simulink model "simulink_group8_2_serial_"  (R2020a)
settings: Solver=FixedStepAuto  StartTime=0.0  StopTime=40  FixedStep=1e-3  RelTol=1e-3  EnableMultiTasking=on
undefined symbols (not defined in the file): A0, A1, D0, D1, D10, D11, D12, D13, D2, D3, D4, D5, D6, D7, D8, D9, magnitude, PTA0, PTA1, PTA2, PTB2, PTB23, PTB3, PTB9, PTC16, PTC17, PTC2, PTC3, PTC4, PTD0, PTD1, PTD2, PTD3
libraries: frdmk64flib x20, etargetslib x10, simulink x4
settings Model: ExtModeTrigDuration=5  Creator=namby  LastModifiedBy=bacTh
settings SolverCC: AutoInsertRateTranBlk=on
settings OptimizationCC: EnhancedBackFolding=on  PassReuseOutputArgsAs=Individual arguments  ZeroExternalMemoryAtStartup=off  ZeroInternalMemoryAtStartup=off  MaxStackSize=64  OptimizeBlockOrder=speed  DifferentSizesBufferReuse=on  OptimizationCustomize=off  EfficientTunableParamExpr=on
settings DebuggingCC: ParameterTunabilityLossMsg=error
settings HardwareCC: ProdBitPerPointer=32  ProdBitPerSizeT=32  ProdBitPerPtrDiffT=32  ProdLargestAtomicInteger=Long  ProdLargestAtomicFloat=Double  ProdWordSize=32  ProdHWDeviceType=ARM Compatible->ARM Cortex
settings SFSimCC: MATLABDynamicMemAlloc=off
settings RTWCC: SystemTargetFile=ert.tlc  HardwareBoard=NXP FRDM-K64F  TemplateMakefile=ert_default_tmf  Toolchain=GNU Tools for ARM Embedded Processors
settings CodeAppCC: ForceParamTrailComments=on  IgnoreCustomStorageClasses=off  OperatorAnnotations=on  SimulinkDataObjDesc=on  SFDataObjDesc=on  InsertBlockDesc=on
settings ConfigComp: CovBoundaryAbsTol=1.0e-5
settings SettingsController: UseSoCProfilerForTargets=0

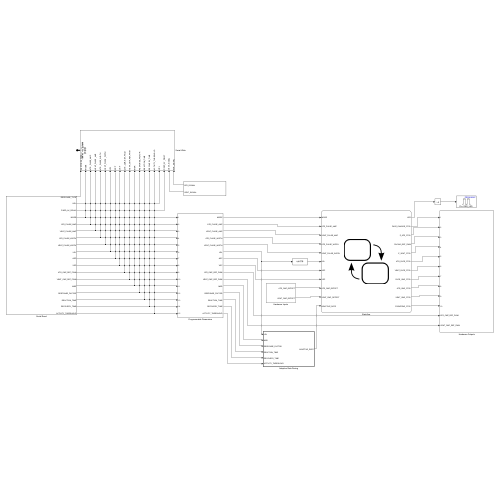
[thumbnail: Simulink's stored preview of the top-level diagram]
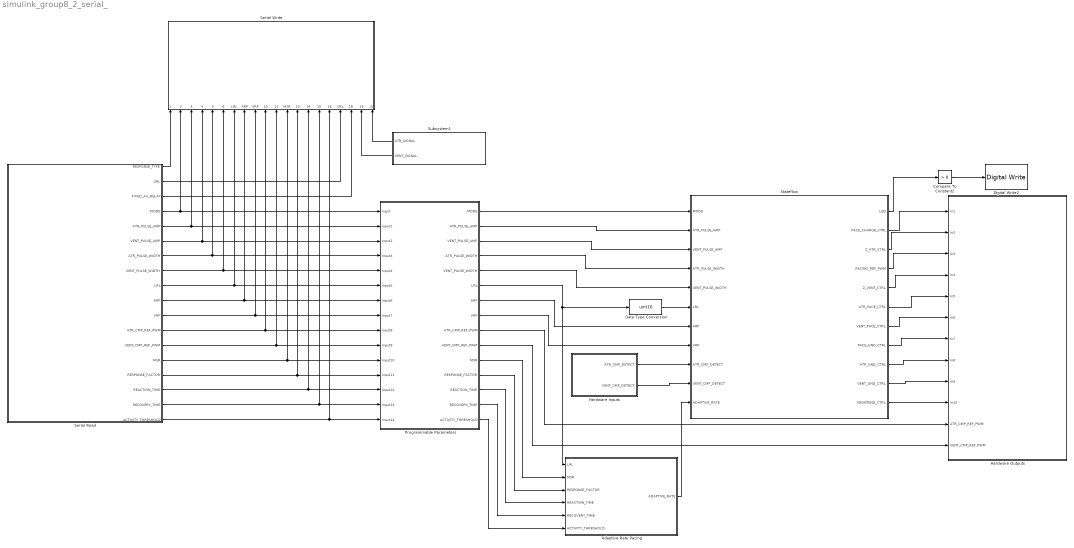
== system simulink_group8_2_serial_ ==
  Adaptive Rate Pacing : Subsystem  TreatAsAtomicUnit=on
  Compare To Constant2 : simulink/Logic and Bit Operations/Compare To Constant  relop=>  const=0  OutDataTypeStr=boolean
  Data Type Conversion : DataTypeConversion  OutDataTypeStr=uint16
  Digital Write2 : frdmk64flib/Digital Write  Whichpin=RED_LED
  Hardware Inputs : Subsystem
  Hardware Outputs : Subsystem
  Programmable Parameters : Subsystem
  Serial Read : Subsystem
  Serial Write : Subsystem
  Stateflow : Stateflow chart  TreatAsAtomicUnit=on
      settings: PortSchema="{\"entries\":[{\"content\":{\"sides\":[{\"content\":{\"connectorIds\":[\"In1\",\"In2\",\"In3\",\"In4\",\"In5\",\"In6\",\"In7\",\"In8\",\"In9\",\"In10\",\"In11\"]},\"type\":\"ConnectorPlacement.EquallySpacedRectSide\",\"uuid\":\"4861ea68-cca1-4690-bebf-db066e06f2bf\"},{\"content\":{\"connectorIds\":[\"Out11\",\"Out1\",\"Out2\",\"Out3\",\"Out4\",\"Out5\",\"Out6\",\"Out7\",\"Out8\",\"Out9\",\"Out10\"],\"side\":\"RIGHT\"},\"type\":\"ConnectorPlacement.EquallySpacedRectSide\",\"uuid\":\"4fa1417b-a578-4dd5-8ec9-8fcbce219e5e\"},{\"content\":{\"side\":\"TOP\"},\"type\":\"ConnectorPlacement.EquallySpacedRectSide\",\"uuid\":\"410f88ae-5c1c-4ed5-8b61-d3fe3ab7a61c\"}]},\"type\":\"ConnectorPlacement.EquallySpacedConnector\",\"uuid\":\"8afcebbc-da82-4773-8c00-253856c85373\"}],\"packageUris\":[\"http://schema.mathworks.com/mf0/Connector/R2020b\"],\"version\":\"1.0\"}"
  Subsystem1 : Subsystem
  wires:
  Programmable Parameters/1(MODE) -> Stateflow/1(MODE)
  Programmable Parameters/2(ATR_PULSE_AMP) -> Stateflow/2(ATR_PULSE_AMP)
  Programmable Parameters/3(VENT_PULSE_AMP) -> Stateflow/3(VENT_PULSE_AMP)
  Programmable Parameters/4(ATR_PULSE_WIDTH) -> Stateflow/4(ATR_PULSE_WIDTH)
  Programmable Parameters/5(VENT_PULSE_WIDTH) -> Stateflow/5(VENT_PULSE_WIDTH)
  Programmable Parameters/6(LRL) -> Adaptive Rate Pacing/1(LRL), Data Type Conversion/1
  Programmable Parameters/7(ARP) -> Stateflow/7(ARP)
  Programmable Parameters/8(VRP) -> Stateflow/8(VRP)
  Hardware Inputs/1(ATR_CMP_DETECT) -> Stateflow/9(ATR_CMP_DETECT)
  Hardware Inputs/2(VENT_CMP_DETECT) -> Stateflow/10(VENT_CMP_DETECT)
  Stateflow/1(PACE_CHARGE_CTRL) -> Hardware Outputs/1(In1)
  Stateflow/2(Z_ATR_CTRL) -> Hardware Outputs/2(In2)
  Stateflow/3(PACING_REF_PWM) -> Hardware Outputs/3(In3)
  Stateflow/4(Z_VENT_CTRL) -> Hardware Outputs/4(In4)
  Stateflow/5(ATR_PACE_CTRL) -> Hardware Outputs/5(In5)
  Stateflow/6(VENT_PACE_CTRL) -> Hardware Outputs/6(In6)
  Stateflow/7(PACE_GND_CTRL) -> Hardware Outputs/7(In7)
  Stateflow/8(ATR_GND_CTRL) -> Hardware Outputs/8(In8)
  Stateflow/9(VENT_GND_CTRL) -> Hardware Outputs/9(In9)
  Stateflow/10(FRONTEND_CTRL) -> Hardware Outputs/10(In10)
  Programmable Parameters/9(ATR_CMP_REF_PWM) -> Hardware Outputs/11(ATR_CMP_REF_PWM)
  Programmable Parameters/10(VENT_CMP_REF_PWM) -> Hardware Outputs/12(VENT_CMP_REF_PWM)
  Adaptive Rate Pacing/1(ADAPTIVE_RATE) -> Stateflow/11(ADAPTIVE_RATE)
  Programmable Parameters/15(ACTIVITY_THRESHOLD) -> Adaptive Rate Pacing/6(ACTIVITY_THRESHOLD)
  Programmable Parameters/13(REACTION_TIME) -> Adaptive Rate Pacing/4(REACTION_TIME)
  Programmable Parameters/14(RECOVERY_TIME) -> Adaptive Rate Pacing/5(RECOVERY_TIME)
  Programmable Parameters/12(RESPONSE_FACTOR) -> Adaptive Rate Pacing/3(RESPONSE_FACTOR)
  Programmable Parameters/11(MSR) -> Adaptive Rate Pacing/2(MSR)
  Subsystem1/1(ATR_SIGNAL) -> Serial Write/20(ATR_SIGNAL)
  Subsystem1/2(VENT_SIGNAL) -> Serial Write/19(VENT_SIGNAL)
  Serial Read/16(REACTION_TIME) -> Serial Write/14(REACTION_TIME), Programmable Parameters/13(Input12)
  Serial Read/5(ATR_PULSE_AMP) -> Programmable Parameters/2(Input1), Serial Write/3(ATR_PULSE_AMP)
  Serial Read/7(ATR_PULSE_WIDTH) -> Programmable Parameters/4(Input3), Serial Write/5(ATR_PULSE_WIDTH)
  Serial Read/4(MODE) -> Programmable Parameters/1(Input), Serial Write/2(MODE)
  Serial Read/17(RECOVERY_TIME) -> Serial Write/15(RECOVERY_TIME), Programmable Parameters/14(Input13)
  Serial Read/8(VENT_PULSE_WIDTH) -> Programmable Parameters/5(Input4), Serial Write/6(VENT_PULSE_WIDTH)
  Serial Read/9(LRL) -> Serial Write/7(LRL), Programmable Parameters/6(Input5)
  Serial Read/6(VENT_PULSE_AMP) -> Programmable Parameters/3(Input2), Serial Write/4(VENT_PULSE_AMP)
  Serial Read/18(ACTIVITY_THRESHOLD) -> Serial Write/16(ACTIVITY_THRESHOLD), Programmable Parameters/15(Input14)
  Serial Read/15(RESPONSE_FACTOR) -> Serial Write/13(RESPONSE_FACTOR), Programmable Parameters/12(Input11)
  Serial Read/11(VRP) -> Serial Write/9(VRP), Programmable Parameters/8(Input7)
  Serial Read/10(ARP) -> Serial Write/8(ARP), Programmable Parameters/7(Input6)
  Serial Read/12(ATR_CMP_REF_PWM) -> Serial Write/10(ATR_CMP_REF_PWM), Programmable Parameters/9(Input8)
  Serial Read/14(MSR) -> Serial Write/12(MSR), Programmable Parameters/11(Input10)
  Serial Read/13(VENT_CMP_REF_PWM) -> Serial Write/11(VENT_CMP_REF_PWM), Programmable Parameters/10(Input9)
  Serial Read/1(RESPONSE_TYPE) -> Serial Write/1(RESPONSE_TYPE)
  Serial Read/2(URL) -> Serial Write/17(URL)
  Serial Read/3(FIXED_AV_DELAY) -> Serial Write/18(FIXED_AV_DELAY)
  Data Type Conversion/1 -> Stateflow/6(LRL)
  Compare To Constant2/1 -> Digital Write2/1
  Stateflow/11(LED) -> Compare To Constant2/1

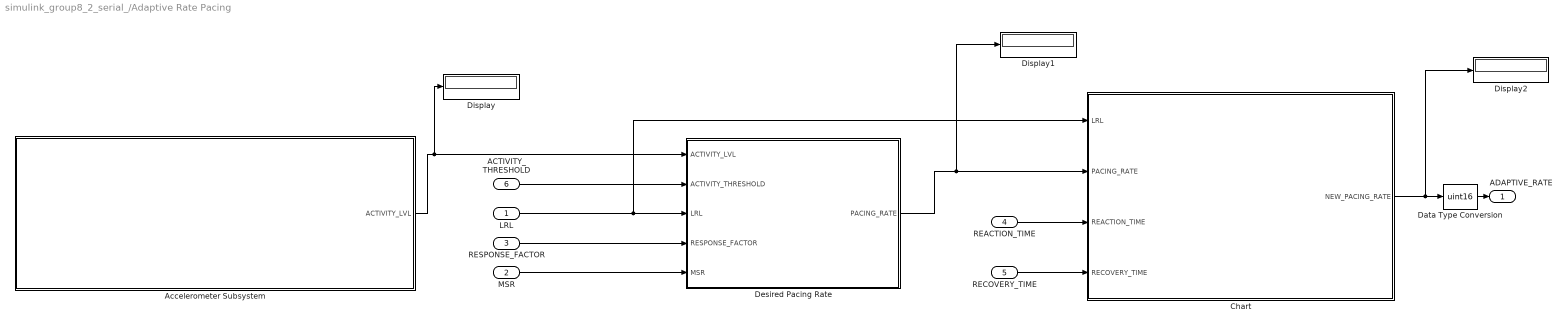
== system simulink_group8_2_serial_/Adaptive Rate Pacing ==
  LRL : Inport
  MSR : Inport  Port=2
  RESPONSE_FACTOR : Inport  Port=3
  REACTION_TIME : Inport  Port=4
  RECOVERY_TIME : Inport  Port=5
  ACTIVITY_THRESHOLD : Inport  Port=6
  Accelerometer Subsystem : Subsystem
  Chart : Stateflow chart  TreatAsAtomicUnit=on
      settings: PortSchema="{\"entries\":[{\"content\":{\"sides\":[{\"content\":{\"connectorIds\":[\"In1\",\"In2\",\"In4\",\"In3\"]},\"type\":\"ConnectorPlacement.EquallySpacedRectSide\",\"uuid\":\"fedab669-afc8-4b81-9e8e-92a87252e5ac\"},{\"content\":{\"connectorIds\":[\"Out1\"],\"side\":\"RIGHT\"},\"type\":\"ConnectorPlacement.EquallySpacedRectSide\",\"uuid\":\"e22eef68-a900-4eb5-a3ef-7284a4069aea\"},{\"content\":{\"side\":\"TOP\"},\"type\":\"ConnectorPlacement.EquallySpacedRectSide\",\"uuid\":\"61fc3a67-93fd-4676-b1c8-d6e22ff2a282\"}]},\"type\":\"ConnectorPlacement.EquallySpacedConnector\",\"uuid\":\"3033053e-278d-4569-b7a9-9d3669d08bbe\"}],\"packageUris\":[\"http://schema.mathworks.com/mf0/Connector/R2020b\"],\"version\":\"1.0\"}"
  Data Type Conversion : DataTypeConversion  OutDataTypeStr=uint16
  Desired Pacing Rate : MATLAB Function  TreatAsAtomicUnit=on
  Display : Display
  Display1 : Display
  Display2 : Display
  ADAPTIVE_RATE : Outport
  wires:
  ACTIVITY_THRESHOLD/1 -> Desired Pacing Rate/2(ACTIVITY_THRESHOLD)
  LRL/1 -> Chart/1(LRL), Desired Pacing Rate/3(LRL)
  RESPONSE_FACTOR/1 -> Desired Pacing Rate/4(RESPONSE_FACTOR)
  MSR/1 -> Desired Pacing Rate/5(MSR)
  Accelerometer Subsystem/1(ACTIVITY_LVL) -> Display/1, Desired Pacing Rate/1(ACTIVITY_LVL)
  Desired Pacing Rate/1(PACING_RATE) -> Display1/1, Chart/2(PACING_RATE)
  REACTION_TIME/1 -> Chart/4(REACTION_TIME)
  RECOVERY_TIME/1 -> Chart/3(RECOVERY_TIME)
  Chart/1(NEW_PACING_RATE) -> Data Type Conversion/1, Display2/1
  Data Type Conversion/1 -> ADAPTIVE_RATE/1

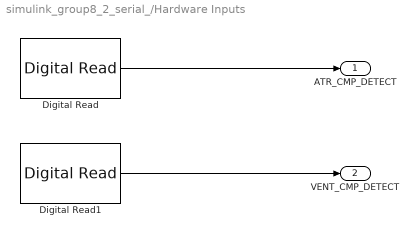
== system simulink_group8_2_serial_/Hardware Inputs ==
  Digital Read : frdmk64flib/Digital Read  Whichpin=PTC16 (D0)  SampleTime=-1
  Digital Read1 : frdmk64flib/Digital Read  Whichpin=PTC17 (D1)  SampleTime=-1
  ATR_CMP_DETECT : Outport
  VENT_CMP_DETECT : Outport  Port=2
  wires:
  Digital Read/1 -> ATR_CMP_DETECT/1
  Digital Read1/1 -> VENT_CMP_DETECT/1

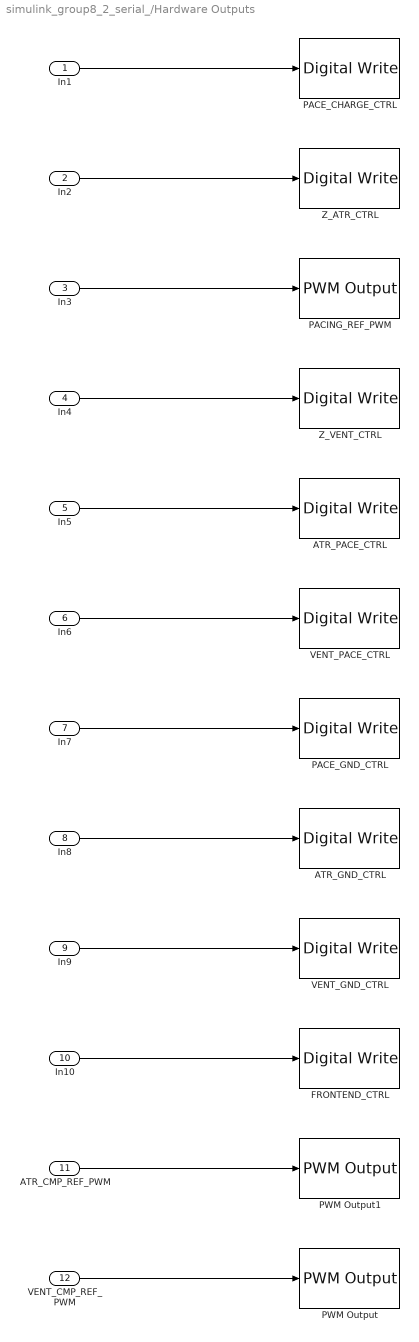
== system simulink_group8_2_serial_/Hardware Outputs ==
  In1 : Inport
  In2 : Inport  Port=2
  In3 : Inport  Port=3
  In4 : Inport  Port=4
  In5 : Inport  Port=5
  In6 : Inport  Port=6
  In7 : Inport  Port=7
  In8 : Inport  Port=8
  In9 : Inport  Port=9
  In10 : Inport  Port=10
  ATR_CMP_REF_PWM : Inport  Port=11
  VENT_CMP_REF_PWM : Inport  Port=12
  ATR_GND_CTRL : frdmk64flib/Digital Write  Whichpin=PTD2 (D11)
  ATR_PACE_CTRL : frdmk64flib/Digital Write  Whichpin=PTA0 (D8)
  FRONTEND_CTRL : frdmk64flib/Digital Write  Whichpin=PTD1 (D13)
  PACE_CHARGE_CTRL : frdmk64flib/Digital Write  Whichpin=PTB9 (D2)
  PACE_GND_CTRL : frdmk64flib/Digital Write  Whichpin=PTD0 (D10)
  PACING_REF_PWM : frdmk64flib/PWM Output  Whichpin=PTA2 (D5)  InitialFrequency=2000  InitialDutyCycle=0
  PWM Output : frdmk64flib/PWM Output  Whichpin=PTA1 (D3)  InitialFrequency=2000  InitialDutyCycle=0
  PWM Output1 : frdmk64flib/PWM Output  Whichpin=PTC2 (D6)  InitialFrequency=2000  InitialDutyCycle=0
  VENT_GND_CTRL : frdmk64flib/Digital Write  Whichpin=PTD3 (D12)
  VENT_PACE_CTRL : frdmk64flib/Digital Write  Whichpin=PTC4 (D9)
  Z_ATR_CTRL : frdmk64flib/Digital Write  Whichpin=PTB23 (D4)
  Z_VENT_CTRL : frdmk64flib/Digital Write  Whichpin=PTC3 (D7)
  wires:
  In1/1 -> PACE_CHARGE_CTRL/1
  In2/1 -> Z_ATR_CTRL/1
  In3/1 -> PACING_REF_PWM/1
  In4/1 -> Z_VENT_CTRL/1
  In5/1 -> ATR_PACE_CTRL/1
  In6/1 -> VENT_PACE_CTRL/1
  In8/1 -> ATR_GND_CTRL/1
  In7/1 -> PACE_GND_CTRL/1
  In10/1 -> FRONTEND_CTRL/1
  In9/1 -> VENT_GND_CTRL/1
  ATR_CMP_REF_PWM/1 -> PWM Output1/1
  VENT_CMP_REF_PWM/1 -> PWM Output/1

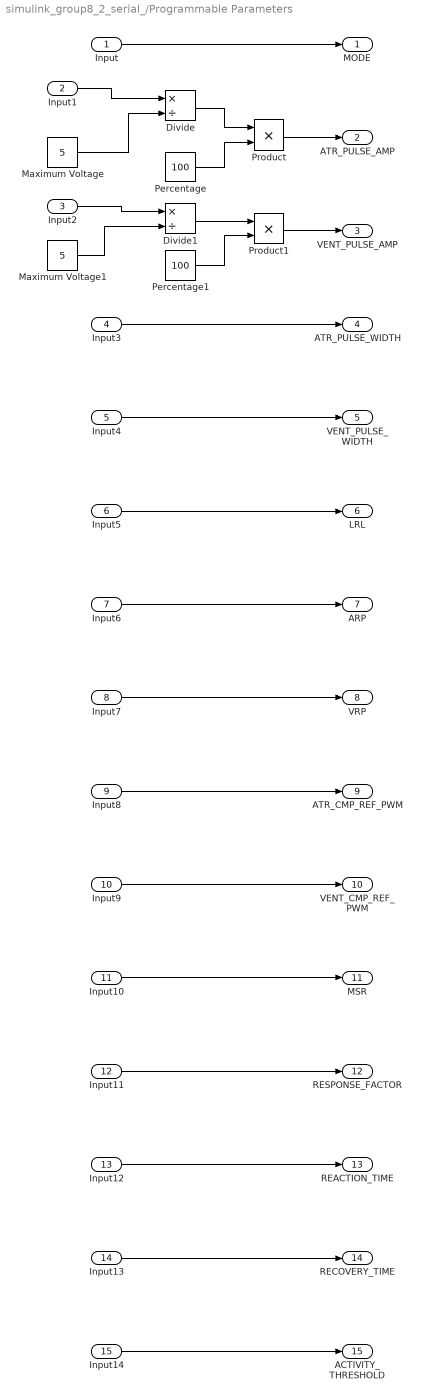
== system simulink_group8_2_serial_/Programmable Parameters ==
  Input : Inport
  Input1 : Inport  Port=2
  Input2 : Inport  Port=3
  Input3 : Inport  Port=4
  Input4 : Inport  Port=5
  Input5 : Inport  Port=6
  Input6 : Inport  Port=7
  Input7 : Inport  Port=8
  Input8 : Inport  Port=9
  Input9 : Inport  Port=10
  Input10 : Inport  Port=11
  Input11 : Inport  Port=12
  Input12 : Inport  Port=13
  Input13 : Inport  Port=14
  Input14 : Inport  Port=15
  Divide : Product  Inputs=*/
  Divide1 : Product  Inputs=*/
  Maximum Voltage : Constant  Value=5
  Maximum Voltage1 : Constant  Value=5
  Percentage : Constant  Value=100
  Percentage1 : Constant  Value=100
  Product : Product
  Product1 : Product
  MODE : Outport
  ATR_PULSE_AMP : Outport  Port=2
  VENT_PULSE_AMP : Outport  Port=3
  ATR_PULSE_WIDTH : Outport  Port=4
  VENT_PULSE_WIDTH : Outport  Port=5
  LRL : Outport  Port=6
  ARP : Outport  Port=7
  VRP : Outport  Port=8
  ATR_CMP_REF_PWM : Outport  Port=9
  VENT_CMP_REF_PWM : Outport  Port=10
  MSR : Outport  Port=11
  RESPONSE_FACTOR : Outport  Port=12
  REACTION_TIME : Outport  Port=13
  RECOVERY_TIME : Outport  Port=14
  ACTIVITY_THRESHOLD : Outport  Port=15
  wires:
  Input/1 -> MODE/1
  Input4/1 -> VENT_PULSE_WIDTH/1
  Input3/1 -> ATR_PULSE_WIDTH/1
  Input5/1 -> LRL/1
  Input6/1 -> ARP/1
  Input7/1 -> VRP/1
  Input8/1 -> ATR_CMP_REF_PWM/1
  Input9/1 -> VENT_CMP_REF_PWM/1
  Maximum Voltage/1 -> Divide/2
  Percentage/1 -> Product/2
  Divide/1 -> Product/1
  Product/1 -> ATR_PULSE_AMP/1
  Percentage1/1 -> Product1/2
  Divide1/1 -> Product1/1
  Maximum Voltage1/1 -> Divide1/2
  Product1/1 -> VENT_PULSE_AMP/1
  Input10/1 -> MSR/1
  Input11/1 -> RESPONSE_FACTOR/1
  Input12/1 -> REACTION_TIME/1
  Input13/1 -> RECOVERY_TIME/1
  Input14/1 -> ACTIVITY_THRESHOLD/1
  Input1/1 -> Divide/1
  Input2/1 -> Divide1/1

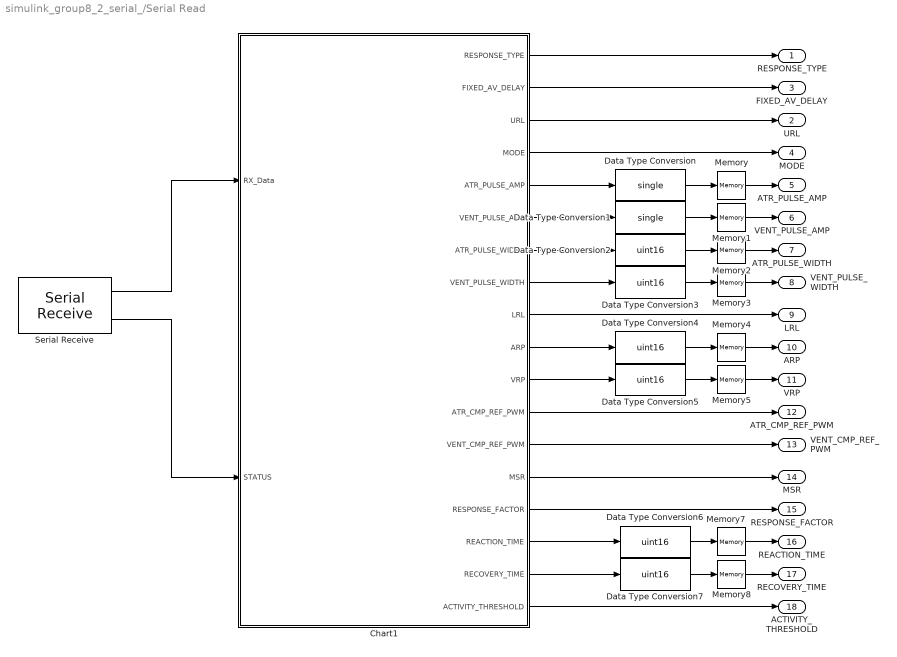
== system simulink_group8_2_serial_/Serial Read ==
  Chart1 : Stateflow chart  TreatAsAtomicUnit=on
      settings: PortSchema="{\"entries\":[{\"content\":{\"sides\":[{\"content\":{\"connectorIds\":[\"In1\",\"In2\"]},\"type\":\"ConnectorPlacement.EquallySpacedRectSide\",\"uuid\":\"1704d51a-e006-419e-ae26-5cef98ca6a68\"},{\"content\":{\"connectorIds\":[\"Out13\",\"Out6\",\"Out14\",\"Out8\",\"Out4\",\"Out16\",\"Out5\",\"Out18\",\"Out7\",\"Out2\",\"Out17\",\"Out3\",\"Out15\",\"Out9\",\"Out12\",\"Out11\",\"Out10\",\"Out1\"],\"side\":\"RIGHT\"},\"type\":\"ConnectorPlacement.EquallySpacedRectSide\",\"uuid\":\"40b8ffc1-f729-40ff-8417-b8a4e5bdb628\"},{\"content\":{\"side\":\"TOP\"},\"type\":\"ConnectorPlacement.EquallySpacedRectSide\",\"uuid\":\"9698f9c2-1891-4130-9240-9b0d7bdea9c8\"},{\"content\":{\"side\":\"BOTTOM\"},\"type\":\"ConnectorPlacement.EquallySpacedRectSide\",\"uuid\":\"9466a883-7f8c-4176-9cbc-8ae72f09588c\"}]},\"type\":\"ConnectorPlacement.EquallySpacedConnector\",\"uuid\":\"58536037-a3ba-413f-8873-efe07892d8f0\"}],\"packageUris\":[\"http://schema.mathworks.com/mf0/Connector/R2020b\"],\"version\":\"1.0\"}"
  Data Type Conversion : DataTypeConversion  OutDataTypeStr=single
  Data Type Conversion1 : DataTypeConversion  OutDataTypeStr=single
  Data Type Conversion{2..7} (6 alike) : DataTypeConversion  OutDataTypeStr=uint16
  Memory{,1..5,7..8} (8 alike) : Memory
  Serial Receive : frdmk64flib/Serial Receive  SCIModule=0  Baudrate=uint32(9600)  Parity=None  StopBits=1  HardwareFlowControl=None  ByteOrder=LittleEndian  DataType=uint8  DataLength=34  BlockingMode=off  OutputStatus=on  SampleTime=0.1
  RESPONSE_TYPE : Outport
  URL : Outport  Port=2
  FIXED_AV_DELAY : Outport  Port=3
  MODE : Outport  Port=4
  ATR_PULSE_AMP : Outport  Port=5
  VENT_PULSE_AMP : Outport  Port=6
  ATR_PULSE_WIDTH : Outport  Port=7
  VENT_PULSE_WIDTH : Outport  Port=8
  LRL : Outport  Port=9
  ARP : Outport  Port=10
  VRP : Outport  Port=11
  ATR_CMP_REF_PWM : Outport  Port=12
  VENT_CMP_REF_PWM : Outport  Port=13
  MSR : Outport  Port=14
  RESPONSE_FACTOR : Outport  Port=15
  REACTION_TIME : Outport  Port=16
  RECOVERY_TIME : Outport  Port=17
  ACTIVITY_THRESHOLD : Outport  Port=18
  wires:
  Chart1/1(ACTIVITY_THRESHOLD) -> ACTIVITY_THRESHOLD/1
  Chart1/17(VRP) -> Data Type Conversion5/1
  Chart1/10(RECOVERY_TIME) -> Data Type Conversion7/1
  Chart1/18(VENT_PULSE_WIDTH) -> Data Type Conversion3/1
  Chart1/6(FIXED_AV_DELAY) -> FIXED_AV_DELAY/1
  Chart1/3(ATR_CMP_REF_PWM) -> ATR_CMP_REF_PWM/1
  Chart1/13(RESPONSE_TYPE) -> RESPONSE_TYPE/1
  Chart1/2(ARP) -> Data Type Conversion4/1
  Chart1/16(VENT_PULSE_AMP) -> Data Type Conversion1/1
  Chart1/12(RESPONSE_FACTOR) -> RESPONSE_FACTOR/1
  Chart1/4(ATR_PULSE_AMP) -> Data Type Conversion/1
  Serial Receive/2 -> Chart1/2(STATUS)
  Chart1/5(ATR_PULSE_WIDTH) -> Data Type Conversion2/1
  Chart1/15(VENT_CMP_REF_PWM) -> VENT_CMP_REF_PWM/1
  Chart1/11(REACTION_TIME) -> Data Type Conversion6/1
  Chart1/7(LRL) -> LRL/1
  Chart1/14(URL) -> URL/1
  Chart1/9(MSR) -> MSR/1
  Chart1/8(MODE) -> MODE/1
  Serial Receive/1 -> Chart1/1(RX_Data)
  Data Type Conversion/1 -> Memory/1
  Data Type Conversion1/1 -> Memory1/1
  Data Type Conversion2/1 -> Memory2/1
  Data Type Conversion3/1 -> Memory3/1
  Data Type Conversion4/1 -> Memory4/1
  Data Type Conversion5/1 -> Memory5/1
  Data Type Conversion6/1 -> Memory7/1
  Data Type Conversion7/1 -> Memory8/1
  Memory/1 -> ATR_PULSE_AMP/1
  Memory1/1 -> VENT_PULSE_AMP/1
  Memory2/1 -> ATR_PULSE_WIDTH/1
  Memory3/1 -> VENT_PULSE_WIDTH/1
  Memory4/1 -> ARP/1
  Memory5/1 -> VRP/1
  Memory7/1 -> REACTION_TIME/1
  Memory8/1 -> RECOVERY_TIME/1

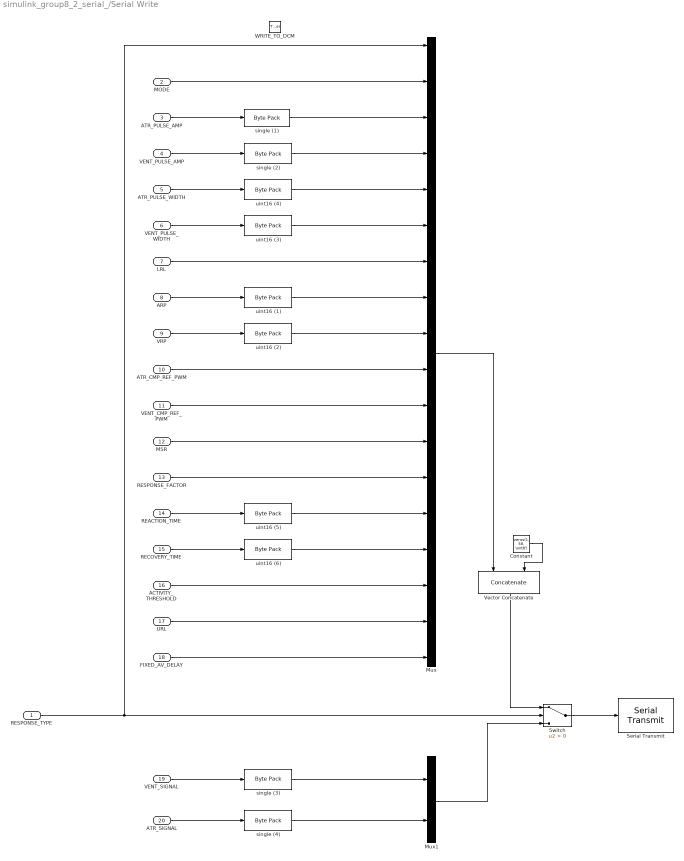
== system simulink_group8_2_serial_/Serial Write ==
  RESPONSE_TYPE : Inport  OutDataTypeStr=uint8
  MODE : Inport  Port=2  OutDataTypeStr=uint8
  ATR_PULSE_AMP : Inport  Port=3  OutDataTypeStr=single
  VENT_PULSE_AMP : Inport  Port=4  OutDataTypeStr=single
  ATR_PULSE_WIDTH : Inport  Port=5  OutDataTypeStr=uint16
  VENT_PULSE_WIDTH : Inport  Port=6  OutDataTypeStr=uint16
  LRL : Inport  Port=7
  ARP : Inport  Port=8  OutDataTypeStr=uint16
  VRP : Inport  Port=9  OutDataTypeStr=uint16
  ATR_CMP_REF_PWM : Inport  Port=10  OutDataTypeStr=uint8
  VENT_CMP_REF_PWM : Inport  Port=11  OutDataTypeStr=uint8
  MSR : Inport  Port=12
  RESPONSE_FACTOR : Inport  Port=13
  REACTION_TIME : Inport  Port=14
  RECOVERY_TIME : Inport  Port=15
  ACTIVITY_THRESHOLD : Inport  Port=16
  URL : Inport  Port=17
  FIXED_AV_DELAY : Inport  Port=18
  VENT_SIGNAL : Inport  Port=19  OutDataTypeStr=single
  ATR_SIGNAL : Inport  Port=20  OutDataTypeStr=single
  WRITE_TO_DCM : TriggerPort  TriggerType=function-call  IsSimulinkFunction=on  FunctionName=WRITE_TO_DCM  VariantControl=Variant
  Constant : Constant  Value=zeros(1, 58, 'uint8')
  Mux : Mux  Inputs=18
  Mux1 : Mux  Inputs=2
  Serial Transmit : frdmk64flib/Serial Transmit  SCIModule=0  Baudrate=uint32(9600)  Parity=None  StopBits=1  HardwareFlowControl=None  ByteOrder=LittleEndian  BlockingMode=off  OutputStatus=off
  Switch : Switch  Criteria=u2 > Threshold
  Vector Concatenate : Concatenate
  single (1) : etargetslib/Byte Pack  datatypes={'single'}  byteAlign=1
  single (2) : etargetslib/Byte Pack  datatypes={'single'}  byteAlign=1
  single (3) : etargetslib/Byte Pack  datatypes={'single'}  byteAlign=1
  single (4) : etargetslib/Byte Pack  datatypes={'single'}  byteAlign=1
  uint16 (1) : etargetslib/Byte Pack  datatypes={'uint16'}  byteAlign=1
  uint16 (2) : etargetslib/Byte Pack  datatypes={'uint16'}  byteAlign=1
  uint16 (3) : etargetslib/Byte Pack  datatypes={'uint16'}  byteAlign=1
  uint16 (4) : etargetslib/Byte Pack  datatypes={'uint16'}  byteAlign=1
  uint16 (5) : etargetslib/Byte Pack  datatypes={'uint16'}  byteAlign=1
  uint16 (6) : etargetslib/Byte Pack  datatypes={'uint16'}  byteAlign=1
  wires:
  RECOVERY_TIME/1 -> uint16 (6)/1
  Mux1/1 -> Switch/3
  single (3)/1 -> Mux1/1
  uint16 (6)/1 -> Mux/15
  uint16 (1)/1 -> Mux/8
  VENT_PULSE_AMP/1 -> single (2)/1
  ACTIVITY_THRESHOLD/1 -> Mux/16
  URL/1 -> Mux/17
  uint16 (4)/1 -> Mux/5
  VRP/1 -> uint16 (2)/1
  MODE/1 -> Mux/2
  single (2)/1 -> Mux/4
  uint16 (2)/1 -> Mux/9
  LRL/1 -> Mux/7
  RESPONSE_TYPE/1 -> Mux/1, Switch/2
  single (4)/1 -> Mux1/2
  ATR_CMP_REF_PWM/1 -> Mux/10
  ATR_PULSE_AMP/1 -> single (1)/1
  single (1)/1 -> Mux/3
  ARP/1 -> uint16 (1)/1
  REACTION_TIME/1 -> uint16 (5)/1
  uint16 (3)/1 -> Mux/6
  VENT_PULSE_WIDTH/1 -> uint16 (3)/1
  uint16 (5)/1 -> Mux/14
  Switch/1 -> Serial Transmit/1
  VENT_SIGNAL/1 -> single (3)/1
  MSR/1 -> Mux/12
  RESPONSE_FACTOR/1 -> Mux/13
  VENT_CMP_REF_PWM/1 -> Mux/11
  ATR_PULSE_WIDTH/1 -> uint16 (4)/1
  ATR_SIGNAL/1 -> single (4)/1
  FIXED_AV_DELAY/1 -> Mux/18
  Constant/1 -> Vector Concatenate/2
  Mux/1 -> Vector Concatenate/1
  Vector Concatenate/1 -> Switch/1

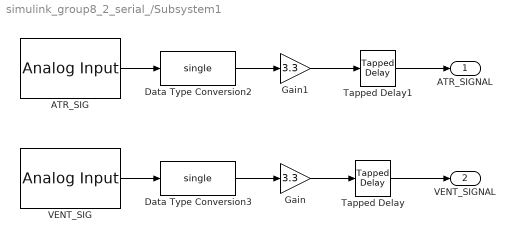
== system simulink_group8_2_serial_/Subsystem1 ==
  ATR_SIG : frdmk64flib/Analog Input  Whichpin=PTB2 (A0)  SampleTime=-1
  Data Type Conversion2 : DataTypeConversion  OutDataTypeStr=single  RndMeth=Nearest
  Data Type Conversion3 : DataTypeConversion  OutDataTypeStr=single  RndMeth=Nearest
  Gain : Gain  Gain=3.3
  Gain1 : Gain  Gain=3.3
  Tapped Delay : simulink/Discrete/Tapped Delay  vinit=0.0  samptime=0.02  NumDelays=10  DelayOrder=Oldest  includeCurrent=on
  Tapped Delay1 : simulink/Discrete/Tapped Delay  vinit=0.0  samptime=0.02  NumDelays=10  DelayOrder=Oldest  includeCurrent=on
  VENT_SIG : frdmk64flib/Analog Input  Whichpin=PTB3 (A1)  SampleTime=-1
  ATR_SIGNAL : Outport
  VENT_SIGNAL : Outport  Port=2
  wires:
  Tapped Delay1/1 -> ATR_SIGNAL/1
  Data Type Conversion2/1 -> Gain1/1
  Gain1/1 -> Tapped Delay1/1
  ATR_SIG/1 -> Data Type Conversion2/1
  VENT_SIG/1 -> Data Type Conversion3/1
  Data Type Conversion3/1 -> Gain/1
  Gain/1 -> Tapped Delay/1
  Tapped Delay/1 -> VENT_SIGNAL/1

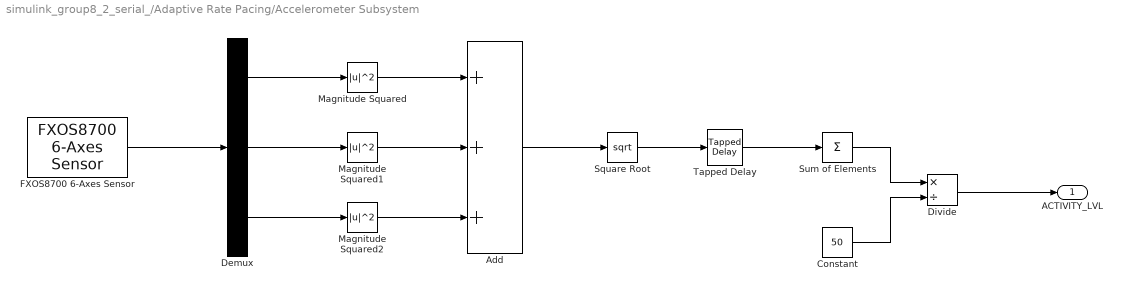
== system simulink_group8_2_serial_/Adaptive Rate Pacing/Accelerometer Subsystem ==
  Add : Sum  Inputs=+++
  Constant : Constant  Value=50
  Demux : Demux  Outputs=3
  Divide : Product  Inputs=*/
  FXOS8700 6-Axes Sensor : frdmk64flib/FXOS8700 6-Axes Sensor  Activesensor=Accelerometer only  ODR=200Hz  HybridODR=400Hz  Accelfullrange=-8g to +8g  SampleTime=0.02
  Magnitude Squared : Math  Operator=magnitude^2  SaturateOnIntegerOverflow=on
  Magnitude Squared1 : Math  Operator=magnitude^2  SaturateOnIntegerOverflow=on
  Magnitude Squared2 : Math  Operator=magnitude^2  SaturateOnIntegerOverflow=on
  Square Root : Sqrt  SaturateOnIntegerOverflow=on
  Sum of Elements : Sum  Inputs=+
  Tapped Delay : simulink/Discrete/Tapped Delay  vinit=0.0  samptime=0.02  NumDelays=50  DelayOrder=Oldest  includeCurrent=off
  ACTIVITY_LVL : Outport
  wires:
  Tapped Delay/1 -> Sum of Elements/1
  Sum of Elements/1 -> Divide/1
  Demux/3 -> Magnitude Squared2/1
  Demux/1 -> Magnitude Squared/1
  Constant/1 -> Divide/2
  FXOS8700 6-Axes Sensor/1 -> Demux/1
  Add/1 -> Square Root/1
  Square Root/1 -> Tapped Delay/1
  Magnitude Squared2/1 -> Add/3
  Magnitude Squared/1 -> Add/1
  Demux/2 -> Magnitude Squared1/1
  Magnitude Squared1/1 -> Add/2
  Divide/1 -> ACTIVITY_LVL/1

== stateflow chart simulink_group8_2_serial_/Adaptive Rate Pacing/Chart ==
  state INIT
    entry:
    NEW_PACING_RATE = LRL
  state RISE
    entry:
    NEW_PACING_RATE = NEW_PACING_RATE + RISE
  state FALL
    entry:
    NEW_PACING_RATE = NEW_PACING_RATE - FALL
  state CALC_STANDBY
    entry:
    if (PACING_RATE > NEW_PACING_RATE)
    RISE = (double(PACING_RATE) - double(NEW_PACING_RATE)) / (double(REACTION_TIME) / double(60));
    FALL = 0;
    elseif (PACING_RATE < NEW_PACING_RATE)
    FALL = (double(NEW_PACING_RATE) - double(PACING_RATE)) / double(RECOVERY_TIME);
    RISE = 0;
    else
    RISE = 0;
    FALL = 0;
    end
  (default) -> INIT
  INIT -> CALC_STANDBY
  FALL -> CALC_STANDBY : after(1000,msec)
  RISE -> CALC_STANDBY : after(1000,msec)
  CALC_STANDBY -> FALL [order 2] : [NEW_PACING_RATE > PACING_RATE]
  CALC_STANDBY -> RISE [order 1] : [NEW_PACING_RATE < PACING_RATE]
  data: LRL input; PACING_RATE input; RECOVERY_TIME input; NEW_PACING_RATE output; RISE local; FALL local; REACTION_TIME input

== stateflow chart simulink_group8_2_serial_/Serial Read/Chart1 ==
  state SET_PARAMS
    entry:
    %Set DCM params
    RESPONSE_TYPE = RX_Data(3);
    MODE = RX_Data(4);
    temp16 = uint16(RX_Data(5)) + bitshift(uint16(RX_Data(6)), 8);
    ARP = double(temp16);
    temp16 = uint16(RX_Data(7)) + bitshift(uint16(RX_Data(8)), 8);
    VRP = double(temp16);
    temp_u32 = uint32(RX_Data(9)) + bitshift(uint32(RX_Data(10)), 8) + bitshift(uint32(RX_Data(11)), 16) + bitshift(uint32(RX_Data(12)), 24);
    ATR_PULSE_AMP = double(typecast(temp_u32, 'single'));
    temp_u32 = uint32(RX_Data(13)) + bitshift(uint32(RX_Data(14)), 8) + bitshift(uint32(RX_Data(15)), 16) + bitshift(uint32(RX_Data(16)), 24);
    VENT_PULSE_AMP = double(typecast(temp_u32, 'single'));
    temp16 = uint16(RX_Data(17)) + bitshift(uint16(RX_Data(18)), 8);
    ATR_PULSE_WIDTH = double(temp16);
    temp16 = uint16(RX_Data(19)) + bitshift(uint16(RX_Data(20)), 8);
    VENT_PULSE_WIDTH = double(temp16);
    ATR_CMP_REF_PWM = RX_Data(22);
    VENT_CMP_REF_PWM = RX_Data(23);
    temp16 = uint16(RX_Data(24)) + bitshift(uint16(RX_Data(25)), 8);
    REACTION_TIME = double(temp16);
    temp16 = uint16(RX_Data(26)) + bitshift(uint16(RX_Data(27)), 8);
    RECOVERY_TIME = double(temp16);
    FIXED_AV_DELAY = RX_Data(29);
    RESPONSE_FACTOR = RX_Data(30);
    ACTIVITY_THRESHOLD = RX_Data(31);
    LRL = RX_Data(32);
    URL = RX_Data(33);
    MSR = RX_Data(34);
    % Return Parameters
    WRITE_TO_DCM()
  state INIT
    entry:
    %Default params
    RESPONSE_TYPE = 1
    % final is 7
    MODE = 1
    ARP = 250
    VRP = 320
    % final is 3
    ATR_PULSE_AMP = 3
    VENT_PULSE_AMP = 3
    ATR_PULSE_WIDTH = 10
    VENT_PULSE_WIDTH = 10
    % final is 62/65
    ATR_CMP_REF_PWM = 62
    VENT_CMP_REF_PWM = 65
    REACTION_TIME = 30
    RECOVERY_TIME = 5
    FIXED_AV_DELAY = 250
    RESPONSE_FACTOR = 8
    ACTIVITY_THRESHOLD = 1
    LRL = 60
    URL = 120
    MSR = 120
  state STANDBY
    %Waiting for DCM
  state ECHO_PARAMS
    entry:
    WRITE_TO_DCM()
  SET_PARAMS -> STANDBY
  (default) -> INIT
  (junction 7) -> STANDBY [order 2]
  INIT -> STANDBY
  STANDBY -> (junction 7) : [STATUS == 0]
  (junction 7) -> (junction 12) [order 1] : [RX_Data(1) == hex2dec('16')]
  (junction 12) -> SET_PARAMS [order 1] : [RX_Data(2) == hex2dec('55')]
  (junction 12) -> ECHO_PARAMS [order 2] : [RX_Data(2) == hex2dec('22')]
  ECHO_PARAMS -> STANDBY
  data: RX_Data input uint8 size=34; STATUS input size=1; ACTIVITY_THRESHOLD output; ARP output; ATR_CMP_REF_PWM output; ATR_PULSE_AMP output; ATR_PULSE_WIDTH output; FIXED_AV_DELAY output; LRL output; MODE output; MSR output; RECOVERY_TIME output; REACTION_TIME output; RESPONSE_FACTOR output; RESPONSE_TYPE output; URL output; VENT_CMP_REF_PWM output; VENT_PULSE_AMP output; VRP output; VENT_PULSE_WIDTH output; temp16 local uint16 size=1; temp_u32 local

== stateflow chart simulink_group8_2_serial_/Stateflow ==
  state DEFAULT_STATE
    entry:
    FRONTEND_CTRL = 0
  state AOOR
    state STATE_2
      %Atrium Pacing
      PACE_CHARGE_CTRL = 0
      PACE_GND_CTRL = 1
      ATR_PACE_CTRL = 1
      ATR_GND_CTRL = 0
      Z_ATR_CTRL = 0
      Z_VENT_CTRL = 0
      VENT_GND_CTRL = 0
      VENT_PACE_CTRL = 0
      LED = 1
    state STATE_1
      %Charging primary capacitor (C22)
      ATR_PACE_CTRL = 0
      VENT_PACE_CTRL = 0
      PACING_REF_PWM = ATR_PULSE_AMP
      PACE_CHARGE_CTRL = 1
      %
      %Discharging blocking capacitor (C21)
      PACE_GND_CTRL = 1
      VENT_PACE_CTRL = 0
      Z_ATR_CTRL = 0
      Z_VENT_CTRL = 0
      ATR_PACE_CTRL = 0
      ATR_GND_CTRL = 1
      VENT_GND_CTRL = 0
      LED = 0
    (default) -> AOOR.STATE_1
    AOOR.STATE_1 -> AOOR.STATE_2 : [after((60000/ADAPTIVE_RATE) - ATR_PULSE_WIDTH, msec)]
    AOOR.STATE_2 -> AOOR.STATE_1 : [after(ATR_PULSE_WIDTH, msec)]
  state AOO
    state STATE_1
      %Charging primary capacitor (C22)
      ATR_PACE_CTRL = 0
      VENT_PACE_CTRL = 0
      PACING_REF_PWM = ATR_PULSE_AMP
      PACE_CHARGE_CTRL = 1
      %
      %Discharging blocking capacitor (C21)
      PACE_GND_CTRL = 1
      VENT_PACE_CTRL = 0
      Z_ATR_CTRL = 0
      Z_VENT_CTRL = 0
      ATR_PACE_CTRL = 0
      ATR_GND_CTRL = 1
      VENT_GND_CTRL = 0
      LED = 0
    state STATE_2
      %Atrium Pacing
      PACE_CHARGE_CTRL = 0
      PACE_GND_CTRL = 1
      ATR_PACE_CTRL = 1
      ATR_GND_CTRL = 0
      Z_ATR_CTRL = 0
      Z_VENT_CTRL = 0
      VENT_GND_CTRL = 0
      VENT_PACE_CTRL = 0
      LED = 1
    (default) -> AOO.STATE_1
    AOO.STATE_1 -> AOO.STATE_2 : [after((60000/LRL) - ATR_PULSE_WIDTH, msec)]
    AOO.STATE_2 -> AOO.STATE_1 : [after(ATR_PULSE_WIDTH, msec)]
  state VOOR
    state STATE_1
      %Charging primary capacitor (C22)
      ATR_PACE_CTRL = 0
      VENT_PACE_CTRL = 0
      PACING_REF_PWM = VENT_PULSE_AMP
      PACE_CHARGE_CTRL = 1
      %
      %Discharging blocking capacitor (C21)
      PACE_GND_CTRL = 1
      VENT_PACE_CTRL = 0
      Z_ATR_CTRL = 0
      Z_VENT_CTRL = 0
      ATR_PACE_CTRL = 0
      ATR_GND_CTRL = 0
      VENT_GND_CTRL = 1
      LED = 0
    state STATE_2
      %Ventricular Pacing
      PACE_CHARGE_CTRL = 0
      PACE_GND_CTRL = 1
      ATR_PACE_CTRL = 0
      ATR_GND_CTRL = 0
      Z_ATR_CTRL = 0
      Z_VENT_CTRL = 0
      VENT_GND_CTRL = 0
      VENT_PACE_CTRL = 1
      LED = 1
    (default) -> VOOR.STATE_1
    VOOR.STATE_1 -> VOOR.STATE_2 : [after((60000/ADAPTIVE_RATE) - VENT_PULSE_WIDTH, msec)]
    VOOR.STATE_2 -> VOOR.STATE_1 : [after(VENT_PULSE_WIDTH, msec)]
  state VOO
    state STATE_1
      %Charging primary capacitor (C22)
      ATR_PACE_CTRL = 0
      VENT_PACE_CTRL = 0
      PACING_REF_PWM = VENT_PULSE_AMP
      PACE_CHARGE_CTRL = 1
      %
      %Discharging blocking capacitor (C21)
      PACE_GND_CTRL = 1
      VENT_PACE_CTRL = 0
      Z_ATR_CTRL = 0
      Z_VENT_CTRL = 0
      ATR_PACE_CTRL = 0
      ATR_GND_CTRL = 0
      VENT_GND_CTRL = 1
      LED = 0
    state STATE_2
      %Ventricular Pacing
      PACE_CHARGE_CTRL = 0
      PACE_GND_CTRL = 1
      ATR_PACE_CTRL = 0
      ATR_GND_CTRL = 0
      Z_ATR_CTRL = 0
      Z_VENT_CTRL = 0
      VENT_GND_CTRL = 0
      VENT_PACE_CTRL = 1
      LED = 1
    (default) -> VOO.STATE_1
    VOO.STATE_1 -> VOO.STATE_2 : [after((60000/LRL) - VENT_PULSE_WIDTH, msec)]
    VOO.STATE_2 -> VOO.STATE_1 : [after(VENT_PULSE_WIDTH, msec)]
  state AAIR
    state ATR_SENSE
      entry:
      %
      %Charging primary capacitor (C22)
      ATR_PACE_CTRL = 0
      VENT_PACE_CTRL = 0
      PACING_REF_PWM = ATR_PULSE_AMP
      PACE_CHARGE_CTRL = 1
      %
      %Discharging blocking capacitor (C21)
      PACE_GND_CTRL = 1
      VENT_PACE_CTRL = 0
      Z_ATR_CTRL = 0
      Z_VENT_CTRL = 0
      ATR_PACE_CTRL = 0
      ATR_GND_CTRL = 1
      VENT_GND_CTRL = 0
      LED = 0
    state STATE_1
      entry:
      %Enable sensing
      FRONTEND_CTRL = 1
      %
      %Charging primary capacitor (C22)
      ATR_PACE_CTRL = 0
      VENT_PACE_CTRL = 0
      PACING_REF_PWM = ATR_PULSE_AMP
      PACE_CHARGE_CTRL = 1
      %
      %Discharging blocking capacitor (C21)
      PACE_GND_CTRL = 1
      VENT_PACE_CTRL = 0
      Z_ATR_CTRL = 0
      Z_VENT_CTRL = 0
      ATR_PACE_CTRL = 0
      ATR_GND_CTRL = 1
      VENT_GND_CTRL = 0
      LED = 0
    state STATE_2
      entry:
      %Atrium Pacing
      PACE_CHARGE_CTRL = 0
      PACE_GND_CTRL = 1
      ATR_PACE_CTRL = 1
      ATR_GND_CTRL = 0
      Z_ATR_CTRL = 0
      Z_VENT_CTRL = 0
      VENT_GND_CTRL = 0
      VENT_PACE_CTRL = 0
      LED = 1
    AAIR.STATE_2 -> AAIR.ATR_SENSE : after(ATR_PULSE_WIDTH, msec)
    AAIR.STATE_1 -> AAIR.ATR_SENSE [order 1] : [ATR_CMP_DETECT == 1]
    (default) -> AAIR.STATE_1
    AAIR.ATR_SENSE -> AAIR.STATE_1 : after(ARP,msec)
    AAIR.STATE_1 -> AAIR.STATE_2 [order 2] : after((60000/ADAPTIVE_RATE) - ATR_PULSE_WIDTH - ARP, msec)[ATR_CMP_DETECT == 0]
  state AAI
    state ATR_SENSE
      entry:
      %
      %Charging primary capacitor (C22)
      ATR_PACE_CTRL = 0
      VENT_PACE_CTRL = 0
      PACING_REF_PWM = ATR_PULSE_AMP
      PACE_CHARGE_CTRL = 1
      %
      %Discharging blocking capacitor (C21)
      PACE_GND_CTRL = 1
      VENT_PACE_CTRL = 0
      Z_ATR_CTRL = 0
      Z_VENT_CTRL = 0
      ATR_PACE_CTRL = 0
      ATR_GND_CTRL = 1
      VENT_GND_CTRL = 0
      LED = 0
    state STATE_1
      entry:
      %Enable sensing
      FRONTEND_CTRL = 1
      %
      %Charging primary capacitor (C22)
      ATR_PACE_CTRL = 0
      VENT_PACE_CTRL = 0
      PACING_REF_PWM = ATR_PULSE_AMP
      PACE_CHARGE_CTRL = 1
      %
      %Discharging blocking capacitor (C21)
      PACE_GND_CTRL = 1
      VENT_PACE_CTRL = 0
      Z_ATR_CTRL = 0
      Z_VENT_CTRL = 0
      ATR_PACE_CTRL = 0
      ATR_GND_CTRL = 1
      VENT_GND_CTRL = 0
      LED = 0
    state STATE_2
      entry:
      %Atrium Pacing
      PACE_CHARGE_CTRL = 0
      PACE_GND_CTRL = 1
      ATR_PACE_CTRL = 1
      ATR_GND_CTRL = 0
      Z_ATR_CTRL = 0
      Z_VENT_CTRL = 0
      VENT_GND_CTRL = 0
      VENT_PACE_CTRL = 0
      LED = 1
    AAI.STATE_1 -> AAI.ATR_SENSE [order 1] : [ATR_CMP_DETECT == 1]
    AAI.STATE_2 -> AAI.ATR_SENSE : after(ATR_PULSE_WIDTH, msec)
    (default) -> AAI.STATE_1
    AAI.ATR_SENSE -> AAI.STATE_1 : after(ARP,msec)
    AAI.STATE_1 -> AAI.STATE_2 [order 2] : after((60000/LRL) - ATR_PULSE_WIDTH - ARP, msec)[ATR_CMP_DETECT == 0]
  state VVIR
    state VENT_SENSE
      entry:
      %Charging primary capacitor (C22)
      ATR_PACE_CTRL = 0
      VENT_PACE_CTRL = 0
      PACING_REF_PWM = VENT_PULSE_AMP
      PACE_CHARGE_CTRL = 1
      %
      %Discharging blocking capacitor (C21)
      PACE_GND_CTRL = 1
      VENT_PACE_CTRL = 0
      Z_ATR_CTRL = 0
      Z_VENT_CTRL = 0
      ATR_PACE_CTRL = 0
      ATR_GND_CTRL = 0
      VENT_GND_CTRL = 1
      LED = 0
    state STATE_1
      entry:
      %Enable Sensing
      FRONTEND_CTRL = 1
      %
      %Charging primary capacitor (C22)
      ATR_PACE_CTRL = 0
      VENT_PACE_CTRL = 0
      PACING_REF_PWM = VENT_PULSE_AMP
      PACE_CHARGE_CTRL = 1
      %
      %Discharging blocking capacitor (C21)
      PACE_GND_CTRL = 1
      VENT_PACE_CTRL = 0
      Z_ATR_CTRL = 0
      Z_VENT_CTRL = 0
      ATR_PACE_CTRL = 0
      ATR_GND_CTRL = 0
      VENT_GND_CTRL = 1
      LED = 0
    state STATE_2
      %Ventricular Pacing
      PACE_CHARGE_CTRL = 0
      PACE_GND_CTRL = 1
      ATR_PACE_CTRL = 0
      ATR_GND_CTRL = 0
      Z_ATR_CTRL = 0
      Z_VENT_CTRL = 0
      VENT_GND_CTRL = 0
      VENT_PACE_CTRL = 1
      LED = 1
    VVIR.STATE_1 -> VVIR.VENT_SENSE [order 1] : [VENT_CMP_DETECT==1]
    VVIR.STATE_2 -> VVIR.VENT_SENSE : after(VENT_PULSE_WIDTH,msec)
    (default) -> VVIR.STATE_1
    VVIR.VENT_SENSE -> VVIR.STATE_1 : after(VRP,msec)
    VVIR.STATE_1 -> VVIR.STATE_2 [order 2] : after((60000/ADAPTIVE_RATE) - VENT_PULSE_WIDTH - VRP, msec)[VENT_CMP_DETECT == 0]
  state VVI
    state VENT_SENSE
      entry:
      %Charging primary capacitor (C22)
      ATR_PACE_CTRL = 0
      VENT_PACE_CTRL = 0
      PACING_REF_PWM = VENT_PULSE_AMP
      PACE_CHARGE_CTRL = 1
      %
      %Discharging blocking capacitor (C21)
      PACE_GND_CTRL = 1
      VENT_PACE_CTRL = 0
      Z_ATR_CTRL = 0
      Z_VENT_CTRL = 0
      ATR_PACE_CTRL = 0
      ATR_GND_CTRL = 0
      VENT_GND_CTRL = 1
      LED = 0
    state STATE_1
      entry:
      %Enable Sensing
      FRONTEND_CTRL = 1
      %
      %Charging primary capacitor (C22)
      ATR_PACE_CTRL = 0
      VENT_PACE_CTRL = 0
      PACING_REF_PWM = VENT_PULSE_AMP
      PACE_CHARGE_CTRL = 1
      %
      %Discharging blocking capacitor (C21)
      PACE_GND_CTRL = 1
      VENT_PACE_CTRL = 0
      Z_ATR_CTRL = 0
      Z_VENT_CTRL = 0
      ATR_PACE_CTRL = 0
      ATR_GND_CTRL = 0
      VENT_GND_CTRL = 1
      LED = 0
    state STATE_2
      %Ventricular Pacing
      PACE_CHARGE_CTRL = 0
      PACE_GND_CTRL = 1
      ATR_PACE_CTRL = 0
      ATR_GND_CTRL = 0
      Z_ATR_CTRL = 0
      Z_VENT_CTRL = 0
      VENT_GND_CTRL = 0
      VENT_PACE_CTRL = 1
      LED = 1
    VVI.STATE_1 -> VVI.VENT_SENSE [order 1] : [VENT_CMP_DETECT==1]
    VVI.STATE_2 -> VVI.VENT_SENSE : after(VENT_PULSE_WIDTH,msec)
    (default) -> VVI.STATE_1
    VVI.VENT_SENSE -> VVI.STATE_1 : after(VRP,msec)
    VVI.STATE_1 -> VVI.STATE_2 [order 2] : after((60000/LRL) - VENT_PULSE_WIDTH - VRP, msec)[VENT_CMP_DETECT == 0]
  (default) -> DEFAULT_STATE
  DEFAULT_STATE -> AOOR [order 5] : [MODE == 5]
  DEFAULT_STATE -> AOO [order 1] : [MODE==1]
  AOOR -> DEFAULT_STATE : [MODE ~= 5]
  AOO -> DEFAULT_STATE : [MODE~=1]
  DEFAULT_STATE -> VOOR [order 6] : [MODE == 6]
  DEFAULT_STATE -> VOO [order 2] : [MODE==2]
  VOOR -> DEFAULT_STATE : [MODE ~= 6]
  VOO -> DEFAULT_STATE : [MODE~=2]
  DEFAULT_STATE -> AAIR [order 7] : [MODE == 7]
  DEFAULT_STATE -> AAI [order 3] : [MODE==3]
  AAIR -> DEFAULT_STATE : [MODE ~= 7]
  AAI -> DEFAULT_STATE : [MODE~=3]
  DEFAULT_STATE -> VVIR [order 8] : [MODE == 8]
  DEFAULT_STATE -> VVI [order 4] : [MODE==4]
  VVIR -> DEFAULT_STATE : [MODE ~= 8]
  VVI -> DEFAULT_STATE : [MODE~=4]
  data: PACE_CHARGE_CTRL output; Z_ATR_CTRL output; PACING_REF_PWM output; Z_VENT_CTRL output; ATR_PACE_CTRL output; VENT_PACE_CTRL output; PACE_GND_CTRL output; ATR_GND_CTRL output; VENT_GND_CTRL output; FRONTEND_CTRL output; MODE input; ATR_PULSE_AMP input; VENT_PULSE_AMP input; ATR_PULSE_WIDTH input; VENT_PULSE_WIDTH input; LRL input; ARP input; VRP input; ATR_CMP_DETECT input; VENT_CMP_DETECT input; ADAPTIVE_RATE input; LED output

== matlab function simulink_group8_2_serial_/Adaptive Rate Pacing/Desired Pacing Rate ==
  data: ACTIVITY_LVL input; ACTIVITY_THRESHOLD input; LRL input; RESPONSE_FACTOR input; MSR input; PACING_RATE output
function PACING_RATE  = fcn(ACTIVITY_LVL, ACTIVITY_THRESHOLD, LRL, RESPONSE_FACTOR, MSR)
    if (ACTIVITY_LVL <= ACTIVITY_THRESHOLD)
        PACING_RATE = LRL;    
    else
        m = (MSR - LRL)/((ACTIVITY_THRESHOLD + (((1.6 - ACTIVITY_THRESHOLD)/16)*(16-(RESPONSE_FACTOR - 1)))) - ACTIVITY_THRESHOLD);
        b = LRL - (m*(ACTIVITY_THRESHOLD));
        if ((m * ACTIVITY_LVL + b) > MSR)
            PACING_RATE = MSR;
        else
            PACING_RATE = m*ACTIVITY_LVL + b;
        end
    end
